simulink model "EX003_FCHEV"  (R2020b)
settings: Solver=VariableStepAuto  StartTime=0.0  StopTime=20e3  MaxStep=1  RelTol=1e-3
libraries: component_lib x30, pid_lib x2
settings Model: Creator=maxjo65  LastModifiedBy=Max

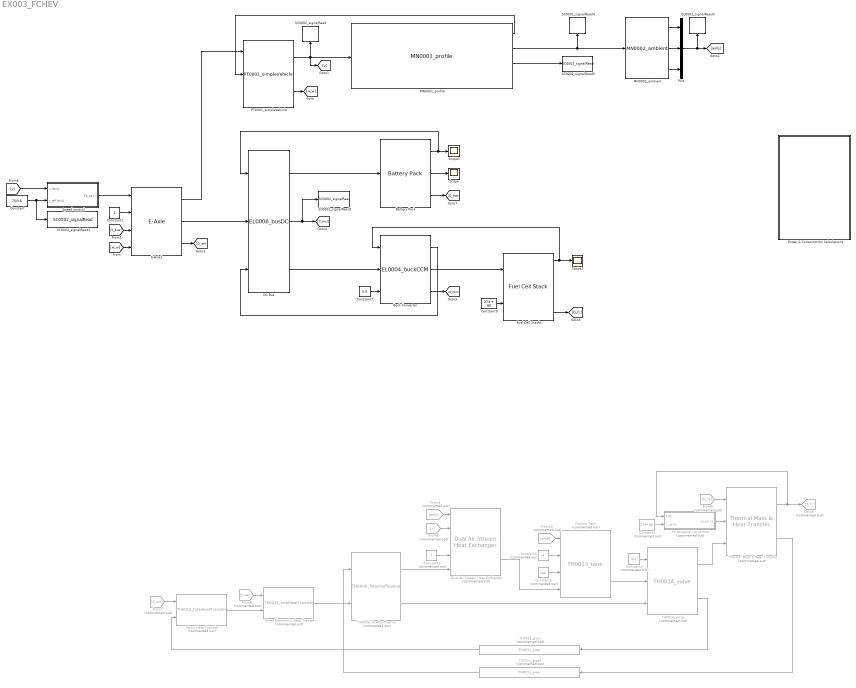
== system EX003_FCHEV ==
  Battery Pack : component_lib/Battery Pack  SOC_0=0.5  Nx=74*10  Ny=6*16  T_bat=273 + 20
  Buck Converter : component_lib/Electrochemistry/EL0004_buckCCM  C=1  L=1  eta=0.9  V_init=400
  Constant : Constant  Value=75/3.6
  Constant1 : Constant
  Constant2 : Constant  Commented=on
  Constant3 : Constant  Commented=on  Value=1/2
  Constant4 : Constant  Commented=on  Value=273+80
  Constant5 : Constant  Commented=on  Value=2e5
  Constant6 : Constant  Commented=on  Value=4
  Constant7 : Constant  Value=0.5
  Constant9 : Constant  Value=273 + 80
  Coolant Tank : component_lib/Thermal Systems/TH0013_tank  Commented=on  V=5e-3
  DC Bus : component_lib/Electrochemistry/EL0006_busDC  C=1  L=912e-9  V_init=340
  Dual Air Stream Heat Exchanger : component_lib/Dual Air Stream Heat Exchanger  Commented=on  HtH=1.1  StS=0.95
  E-Axle1 : component_lib/E-Axle  n=2
  FC temperature control : Subsystem  Commented=on
  From1 : From  Commented=on  GotoTag=v
  From10 : From  Commented=on  GotoTag=amb
  From3 : From  Commented=on  GotoTag=amb
  From7 : From  Commented=on  GotoTag=Q_em
  From8 : From  Commented=on  GotoTag=Q_elec
  From9 : From  Commented=on  GotoTag=Q_fc
  Fuel Cell Stacks : component_lib/Fuel Cell Stack  n=335*2
  Goto8 : Goto  Commented=on  GotoTag=T_fc
  MN0001_profile : component_lib/Mission/MN0001_profile  profile=Munchen.mat  x0=0  N_lookahead=100
  MN0002_ambient : component_lib/Mission/MN0002_ambient  p_0=1.01e5  T_0=273 + 20  RH_0=0.2
  Motor Heat Transfer : component_lib/Thermal Systems/TH0015_totalHeatTransfer  Commented=on  SystemSampleTime=-1  VariantActivationTime=update diagram  Latency=0  AutoFrameSizeCalculation=off
  Mux : Mux  Inputs=3
  PT0001_simpleVehicle : component_lib/Powertrain/PT0001_simpleVehicle  m=40e3  r_w=0.5  A_f=10  C_d=0.5  rho_air=1.225  c_r0=0.0060  c_r1=2.3e-7  gain=600  v0=75/3.6  x0=0
  Power & Consumption Calculations : Subsystem
  Power Electronics Heat Transfer : component_lib/Thermal Systems/TH0015_totalHeatTransfer  Commented=on  SystemSampleTime=-1  VariantActivationTime=update diagram  Latency=0  AutoFrameSizeCalculation=off
  SC0002_signalRead : component_lib/Data & Control/SC0002_signalRead  SigName=velocity
  SC0002_signalRead1 : component_lib/Data & Control/SC0002_signalRead  SigName=busVoltage
  SC0002_signalRead2 : component_lib/Data & Control/SC0002_signalRead  SigName=velocityReference
  SC0002_signalRead3 : component_lib/Data & Control/SC0002_signalRead  SigName=ambient
  SC0002_signalRead4 : component_lib/Data & Control/SC0002_signalRead  SigName=altitude
  SC0002_signalRead5 : component_lib/Data & Control/SC0002_signalRead  SigName=distance
  Scope : Scope
  Scope1 : Scope
  Scope2 : Scope
  Speed control : Subsystem
  TH0006_flowConfluence : component_lib/Thermal Systems/TH0006_flowConfluence  Commented=on  gain=0.01
  TH0011_pipe : component_lib/Thermal Systems/TH0011_pipe  Commented=on  d=3e-2  L=2  T_0=273 + 20  p_0=2e5  W_0=2
  TH0011_pipe1 : component_lib/Thermal Systems/TH0011_pipe  Commented=on  d=3e-2  L=2  T_0=273 + 20  p_0=2e5  W_0=2
  TH0014_valve : component_lib/Thermal Systems/TH0014_valve  Commented=on  d=10e-2  dr=5e-2  C_d=0.9
  Thermal Mass & Heat Transfer : component_lib/Thermal Mass & Heat Transfer  Commented=on  n=335  d=2e-3  L=50e-2  m=150  cp=420  T_0=273 + 20
  wires:
  MN0001_profile/2 -> MN0002_ambient/1, SC0002_signalRead4/1
  Constant/1 -> Speed control/2(v_ref [m/s]), SC0002_signalRead2/1
  PT0001_simpleVehicle/1 -> SC0002_signalRead/1, [v], MN0001_profile/1
  PT0001_simpleVehicle/2 -> [w_w]
  MN0001_profile/1 -> PT0001_simpleVehicle/2
  Mux/1 -> [amb], SC0002_signalRead3/1
  MN0002_ambient/2 -> Mux/2
  MN0002_ambient/1 -> Mux/1
  MN0002_ambient/3 -> Mux/3
  MN0001_profile/3 -> SC0002_signalRead5/1
  Constant5/1 -> Coolant Tank/3
  Constant6/1 -> Coolant Tank/2
  Constant4/1 -> FC temperature control/2(T_ref [K])
  [V_bus] -> E-Axle1/3
  [w_w] -> E-Axle1/4
  [v] -> Speed control/1(v [m/s])
  From1/1 -> Dual Air Stream Heat Exchanger/2
  FC temperature control/1(th_ctrl [-]) -> Thermal Mass & Heat Transfer/2
  Constant2/1 -> Dual Air Stream Heat Exchanger/4
  Battery Pack/1 -> DC Bus/1, Scope1/1
  Speed control/1(Tq_sig [-]) -> E-Axle1/1
  Constant1/1 -> E-Axle1/2
  E-Axle1/1 -> PT0001_simpleVehicle/1
  Motor Heat Transfer/1 -> Power Electronics Heat Transfer/2
  TH0011_pipe/1 -> Motor Heat Transfer/2
  Thermal Mass & Heat Transfer/1 -> FC temperature control/1(T [K]), Goto8/1
  Dual Air Stream Heat Exchanger/2 -> Coolant Tank/4
  From10/1 -> Coolant Tank/1
  From3/1 -> Dual Air Stream Heat Exchanger/1
  Coolant Tank/2 -> TH0014_valve/2
  Constant3/1 -> TH0014_valve/1
  TH0014_valve/1 -> Thermal Mass & Heat Transfer/3
  TH0014_valve/2 -> TH0011_pipe/1
  Power Electronics Heat Transfer/1 -> TH0006_flowConfluence/2
  TH0006_flowConfluence/1 -> Dual Air Stream Heat Exchanger/5
  Thermal Mass & Heat Transfer/2 -> TH0011_pipe1/1
  TH0006_flowConfluence/2 -> TH0014_valve/3
  TH0011_pipe1/1 -> TH0006_flowConfluence/1
  E-Axle1/3 -> [Q_em]
  From7/1 -> Motor Heat Transfer/1
  From8/1 -> Power Electronics Heat Transfer/1
  Fuel Cell Stacks/4 -> [Q_fc]
  From9/1 -> Thermal Mass & Heat Transfer/1
  Battery Pack/3 -> [Q_bat]
  DC Bus/1 -> Battery Pack/1
  DC Bus/2 -> [V_bus], SC0002_signalRead1/1
  Buck Converter/2 -> Fuel Cell Stacks/1
  Buck Converter/1 -> DC Bus/3
  Battery Pack/2 -> Scope/1
  Constant9/1 -> Fuel Cell Stacks/2
  E-Axle1/2 -> DC Bus/2
  Fuel Cell Stacks/1 -> Buck Converter/1, Scope2/1
  Constant7/1 -> Buck Converter/3
  DC Bus/3 -> Buck Converter/2
  Buck Converter/3 -> [Q_buck]

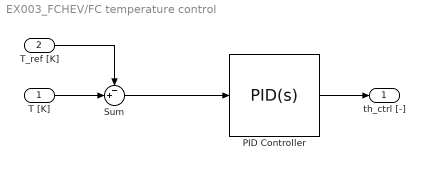
== system EX003_FCHEV/FC temperature control ==
  T [K] : Inport
  T_ref [K] : Inport  Port=2
  PID Controller : pid_lib/PID Controller  Controller=PID  Form=Parallel  TimeDomain=Continuous-time  UseExternalTs=off  SampleTime=-1  IntegratorMethod=Forward Euler  FilterMethod=Forward Euler  ControllerParametersSource=internal  P=1e-2  I=1e-3  D=0  UseFilter=on  N=100  TunerSelectOption=Transfer Function Based (PID Tuner App)  InitialConditionSource=internal  InitialConditionForIntegrator=0  InitialConditionForFilter=0  DifferentiatorICPrevScaledInput=0  ExternalReset=none  TrackingMode=off  Kt=1  LimitOutput=on  SatLimitsSource=internal  UpperSaturationLimit=1  LowerSaturationLimit=0  LinearizeAsGain=on  AntiWindupMode=none  Kb=1  POutMin=[]  POutMax=[]  IOutMin=[]  IOutMax=[]  DOutMin=[]  DOutMax=[]  NOutMin=[]  NOutMax=[]  SumOutMin=[]  SumOutMax=[]  SaturationOutMin=[]  SaturationOutMax=[]  PParamMin=[]  PParamMax=[]  IParamMin=[]  IParamMax=[]  DParamMin=[]  DParamMax=[]  NParamMin=[]  NParamMax=[]  KbParamMin=[]  KbParamMax=[]  KtParamMin=[]  KtParamMax=[]  KbOutMin=[]  KbOutMax=[]  KtOutMin=[]  KtOutMax=[]  IntegratorOutMin=[]  IntegratorOutMax=[]  FilterOutMin=[]  FilterOutMax=[]  SumI1OutMin=[]  SumI1OutMax=[]  SumI2OutMin=[]  SumI2OutMax=[]  SumI3OutMin=[]  SumI3OutMax=[]  SumI4OutMin=[]  SumI4OutMax=[]  SumDOutMin=[]  SumDOutMax=[]  DifferentiatorOutMin=[]  DifferentiatorOutMax=[]  FilterDiffOutCoefMin=[]  FilterDiffOutCoefMax=[]  ReciprocalOutMin=[]  ReciprocalOutMax=[]  SumDenOutMin=[]  SumDenOutMax=[]  SumNumOutMin=[]  SumNumOutMax=[]  DivideOutMin=[]  DivideOutMax=[]  UdiffTsProdOutMin=[]  UdiffTsProdOutMax=[]  NTsProdOutMin=[]  NTsProdOutMax=[]  UintegralTsProdOutMin=[]  UintegralTsProdOutMax=[]  UngainTsProdOutMin=[]  UngainTsProdOutMax=[]  IntegratorContinuousStateAttributes=''  IntegratorStateMustResolveToSignalObject=off  IntegratorRTWStateStorageClass=Auto  FilterContinuousStateAttributes=''  FilterStateMustResolveToSignalObject=off  FilterRTWStateStorageClass=Auto  ParallelPVariant=InternalParameters  IdealPVariant=Disabled  IVariant=InternalParameters  DVariant=InternalParameters  IntegratorVariant=Continuous  SatVariant=Enabled  AWVariant=Passthrough  PCopyVariant=Disabled  TRVariant=Disabled  FdbkBlocksVariant=Forward  IdealPFdbkVariant=Disabled  SatFdbkVariant=Disabled  DerivativeFilterVariant=ContFilter  NVariant=InternalParameters  NCopyVariant=Disabled  FilterICVariant=InternalICsFilter  IntegratorICVariant=InternalICs  ExternalResetVariant=Disabled  TRSumVariant=Passthrough  SumFdbkVariant=Disabled  SumVariant=Sum_PID  TsampFilterVariant=InternalTs  TsampNgainVariant=Passthrough  TsampIntegralVariant=Passthrough  ExternalSaturationOutDataTypeStr=Inherit: Same as second input
  Sum : Sum  Inputs=-+|
  th_ctrl [-] : Outport
  wires:
  PID Controller/1 -> th_ctrl [-]/1
  T_ref [K]/1 -> Sum/1
  T [K]/1 -> Sum/2
  Sum/1 -> PID Controller/1

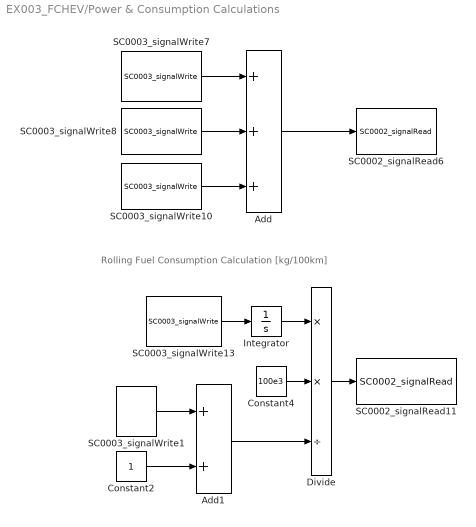
== system EX003_FCHEV/Power & Consumption Calculations ==
  note: Rolling Fuel Consumption Calculation [kg/100km]
  Add : Sum  Inputs=+++
  Add1 : Sum
  Constant2 : Constant
  Constant4 : Constant  Value=100e3
  Divide : Product  Inputs=**/
  Integrator : Integrator
  SC0002_signalRead11 : component_lib/Data & Control/SC0002_signalRead  SigName=fuelConsumption
  SC0002_signalRead6 : component_lib/Data & Control/SC0002_signalRead  SigName=producedPower
  SC0003_signalWrite1 : component_lib/Data & Control/SC0003_signalWrite  SigName=distance
  SC0003_signalWrite10 : component_lib/Data & Control/SC0003_signalWrite  SigName=burnOffPower
  SC0003_signalWrite13 : component_lib/Data & Control/SC0003_signalWrite  SigName=hydrogenFlow
  SC0003_signalWrite7 : component_lib/Data & Control/SC0003_signalWrite  SigName=batteryPower
  SC0003_signalWrite8 : component_lib/Data & Control/SC0003_signalWrite  SigName=fuelCellPower
  wires:
  Integrator/1 -> Divide/1
  SC0003_signalWrite7/1 -> Add/1
  SC0003_signalWrite10/1 -> Add/3
  SC0003_signalWrite1/1 -> Add1/1
  SC0003_signalWrite8/1 -> Add/2
  Add/1 -> SC0002_signalRead6/1
  Add1/1 -> Divide/3
  Constant4/1 -> Divide/2
  Constant2/1 -> Add1/2
  Divide/1 -> SC0002_signalRead11/1
  SC0003_signalWrite13/1 -> Integrator/1

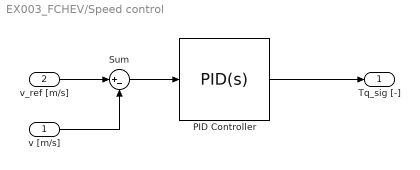
== system EX003_FCHEV/Speed control ==
  v [m/s] : Inport
  v_ref [m/s] : Inport  Port=2
  PID Controller : pid_lib/PID Controller  Controller=PID  Form=Parallel  TimeDomain=Continuous-time  UseExternalTs=off  SampleTime=-1  IntegratorMethod=Forward Euler  FilterMethod=Forward Euler  ControllerParametersSource=internal  P=10  I=1e-1  D=0  UseFilter=on  N=100  TunerSelectOption=Transfer Function Based (PID Tuner App)  InitialConditionSource=internal  InitialConditionForIntegrator=0  InitialConditionForFilter=0  DifferentiatorICPrevScaledInput=0  ExternalReset=none  TrackingMode=off  Kt=1  LimitOutput=on  SatLimitsSource=internal  UpperSaturationLimit=1  LowerSaturationLimit=-1  LinearizeAsGain=on  AntiWindupMode=clamping  Kb=1  POutMin=[]  POutMax=[]  IOutMin=[]  IOutMax=[]  DOutMin=[]  DOutMax=[]  NOutMin=[]  NOutMax=[]  SumOutMin=[]  SumOutMax=[]  SaturationOutMin=[]  SaturationOutMax=[]  PParamMin=[]  PParamMax=[]  IParamMin=[]  IParamMax=[]  DParamMin=[]  DParamMax=[]  NParamMin=[]  NParamMax=[]  KbParamMin=[]  KbParamMax=[]  KtParamMin=[]  KtParamMax=[]  KbOutMin=[]  KbOutMax=[]  KtOutMin=[]  KtOutMax=[]  IntegratorOutMin=[]  IntegratorOutMax=[]  FilterOutMin=[]  FilterOutMax=[]  SumI1OutMin=[]  SumI1OutMax=[]  SumI2OutMin=[]  SumI2OutMax=[]  SumI3OutMin=[]  SumI3OutMax=[]  SumI4OutMin=[]  SumI4OutMax=[]  SumDOutMin=[]  SumDOutMax=[]  DifferentiatorOutMin=[]  DifferentiatorOutMax=[]  FilterDiffOutCoefMin=[]  FilterDiffOutCoefMax=[]  ReciprocalOutMin=[]  ReciprocalOutMax=[]  SumDenOutMin=[]  SumDenOutMax=[]  SumNumOutMin=[]  SumNumOutMax=[]  DivideOutMin=[]  DivideOutMax=[]  UdiffTsProdOutMin=[]  UdiffTsProdOutMax=[]  NTsProdOutMin=[]  NTsProdOutMax=[]  UintegralTsProdOutMin=[]  UintegralTsProdOutMax=[]  UngainTsProdOutMin=[]  UngainTsProdOutMax=[]  IntegratorContinuousStateAttributes=''  IntegratorStateMustResolveToSignalObject=off  IntegratorRTWStateStorageClass=Auto  FilterContinuousStateAttributes=''  FilterStateMustResolveToSignalObject=off  FilterRTWStateStorageClass=Auto  ParallelPVariant=InternalParameters  IdealPVariant=Disabled  IVariant=InternalParameters  DVariant=InternalParameters  IntegratorVariant=Continuous  SatVariant=Enabled  AWVariant=ContClampingParallel  PCopyVariant=Disabled  TRVariant=Disabled  FdbkBlocksVariant=Forward  IdealPFdbkVariant=Disabled  SatFdbkVariant=Disabled  DerivativeFilterVariant=ContFilter  NVariant=InternalParameters  NCopyVariant=Disabled  FilterICVariant=InternalICsFilter  IntegratorICVariant=InternalICs  ExternalResetVariant=Disabled  TRSumVariant=Passthrough  SumFdbkVariant=Disabled  SumVariant=Sum_PID  TsampFilterVariant=InternalTs  TsampNgainVariant=Passthrough  TsampIntegralVariant=Passthrough  ExternalSaturationOutDataTypeStr=Inherit: Same as second input
  Sum : Sum  Inputs=|+-
  Tq_sig [-] : Outport
  wires:
  PID Controller/1 -> Tq_sig [-]/1
  Sum/1 -> PID Controller/1
  v_ref [m/s]/1 -> Sum/1
  v [m/s]/1 -> Sum/2
